simulink model "HIL_Testing_SW_amantest"  (Simulink 7.5)
settings: Solver=ode1  StartTime=0.0  StopTime=Inf  FixedStep=0.001  RelTol=1e-3
PostLoadFcn:
  | , if any(exist('dsrtsu_mdlpostloadfcn', 'file') == [2, 3, 6]), try dsrtsu_mdlpostloadfcn('Execute', bdroot); catch fprintf('Error in PostLoadFcn (dsrtsu_mdlpostloadfcn) for model "%s":\n %s\n', bdroot, lasterr); end, end,
undefined symbols (not defined in the file): CeBSER_Cnt_NumTempAxisPts, ChargeCord, ChargeCord_Control, ChargeToSOCCurr, ChrgCurrLim, CrntSens1Fine, CS_SOCSetPt, CyclerMaxChrgPwr, CyclerMaxDschrgPwr, deltaAhr, Drive_1, Drive_10, Drive_11, Drive_12, Drive_13, Drive_14, Drive_15, Drive_16, Drive_17, Drive_18, Drive_19, Drive_2, Drive_20, Drive_21, Drive_22, Drive_23, Drive_24, Drive_25, Drive_26, Drive_27, Drive_28, Drive_29, Drive_3, Drive_30, Drive_31, Drive_32, Drive_33, Drive_34, Drive_35, Drive_36, Drive_37, Drive_38, Drive_39, Drive_4, Drive_40, Drive_41, Drive_42, Drive_43, Drive_44, Drive_45, Drive_46, Drive_47, Drive_48, Drive_49, Drive_5, Drive_50, Drive_51, Drive_6, Drive_7, Drive_8 ... (+50)
libraries: simulink x129, rtican x50, rti2211sailib x5, rti2211serlib x5, rti2202miolib x3
(part 9 of 23)

== system HIL_Testing_SW_amantest/RX/Read EREV/Read HVEM ==
  Compare To Constant : simulink/Logic and Bit Operations/Compare To Constant  SystemSampleTime=-1  relop=<=  const=0  LogicOutDataTypeMode=uint8  ZeroCross=off
  Current : Subsystem
  Enabled Subsystem : Subsystem  TreatAsAtomicUnit=on
  HV_Battery_Sensed_Output_HV1 : rtican/RTICAN Receive (RX)   SystemSampleTime=-1  Reserved1=[]  Reserved2=[]  Reserved3=[]  Reserved4=[]  SfcnMessage=[]  Msg_Struct=[]  BoardTypeNo=[]  BoardNo=[]  ChannelNo=[]  Parameters=[]  DialogFcn=[]  UnitName=[]  Revision=[]  UnitValues=[]  DSProperties=struct('RTI',struct('Version',uint32(5),'BlockType',struct('isSLSource',uint8(1),'isSLSink',uint8(1),'isHWSource',uint8(0),'isHWSink',uint8(0),'isSetup',uint8(0),'isInline',uint8(1),'isNonInline',uint8(0),'isInterrupt',uint8(0),'isChannelwise',uint8(0)),'IOBoardType','RTICAN','UnitType','MESSAGE','Identifier','RX','DialogType','MSVC','BlockSet','RTICAN','SlaveProcessor','CAN'))  RTIBlockInterface=struct('OutputPortsWidth',int32([1 1 1 1 1 1 1 1 1]),'OutputPortsActive',[1 1 1 1 1 1 1 1 1],'OutputPortsName',{{'HVBSO_Sns2Crnt','HVBSO_Sns1Crnt','HVBSO_BattVltg','HVBSO_Sns2CrntM','HVBSO_Sns1CrntM','HVBSO_BattVltgM','HVBSO_Sns2CrntV','HVBSO_Sns1CrntV','HVBSO_BattVltgV'}},'OutputPortsDataType',{{'SS_DOUBLE','SS_DOUBLE','SS_DOUBLE','SS_DOUBLE','SS_DOUBLE','SS_DOUBLE','SS_DOUBLE','SS_DOUBLE','SS_DOUBLE'}},'OutputPortsLabel',{{'HVBSO_Sns2Crnt','HVBSO_Sns1Crnt','HVBSO_BattVltg','HVBSO_Sns2CrntM','HVBSO_Sns1CrntM','HVBSO_BattVltgM','HVBSO_Sns2CrntV','HVBSO_Sns1CrntV','HVBSO_BattVltgV'}},'OutputPortsLabelMode','ON','InputPortsWidth',int32(0),'InputPortsActive',0,'DialogFcn','rtican_message_interface_gui','BlockDisplay',{{'','center'}},'IconTransparency','on','ParameterTunableNames',{{}},'InitLevel',3,'BlockName',struct('Token',{{'HV_Battery_Sensed_Output_HV'}}),'SampleTime',{{-1}},'TriggerPort',{{'none'}},'EnablePort',{{'none'}})  RTIBlockParameters=struct('BoardTypeNo',{{4302,'OFF',[]}},'BoardNo',{{1,'ON',[1 16]}},'ChannelNo',{{4,'ON',[1 4]}},'Parameters',{{struct('DataFileSupport',struct('DataFileSelectedMaster',1,'DataFileSelectedLocal',1,'DataFileName',['c:\data\databases\6.4.1\globala - hv.dbc|c:\users\hybriderevdomainga\models3x\serialdatabases\v4.4.5(10505)\globala - hvdmx112.dbc|'],'DataFileDate',['04-Jan-2013 08:37:04'],'SelectedFile',['..\databases\8.0.1 (13015)\globala - hv.dbc'],'InterfaceFcn','rtican_dbc_file_parser'),'Options',struct('StatusSelected',0,'TimeSelected',0,'DeltaTimeSelected',0,'BytePortSelected',0,'MessageLengthSelected',0,'TriggerPort',struct('Selected',0,'TriggerType',0),'UserCoding',struct('Selected',0,'InterfaceFile','UserDecodingFile','FcnName','UserDecodeFcn','InportSelected',0,'InportWidth',1,'OutportSelected',0,'OutportWidth',1),'EnablePortSelected',0,'SignalOnPortnameSelected',1,'UseRXService',0),'Message',struct('MsgOnBlocknameSelected',1,'MsgName','HV_Battery_Sensed_Output_HV','MsgIdFormat',0,'MsgId',534,'MsgLength',7,'NumSignals',9,'SampleTime',-1,'Signal',struct('SgnName',{'HVBSO_Sns2Crnt','HVBSO_Sns1Crnt','HVBSO_BattVltg','HVBSO_Sns2CrntM','HVBSO_Sns1CrntM','HVBSO_BattVltgM','HVBSO_Sns2CrntV','HVBSO_Sns1CrntV','HVBSO_BattVltgV'},'SgnStartBit',{0,16,32,44,45,46,47,48,49},'SgnLength',{16,16,12,1,1,1,1,1,1},'ByteLayout',{2,2,2,2,2,2,2,2,2},'Factor',{0.02,0.02,0.125,1,1,1,1,1,1},'Offset',{0,0,0,0,0,0,0,0,0},'SgnComment',{'','','','','','','','',''},'SgnUnit',{'amps','amps','volts','','','','','',''},'Min',{-655.36,-655.36,0,0,0,0,0,0,0},'Max',{655.34,655.34,511.875,1,1,1,1,1,1},'SgnType',{0,0,0,0,0,0,0,0,0},'SLDataType',{'SS_DOUBLE','SS_DOUBLE','SS_DOUBLE','SS_DOUBLE','SS_DOUBLE','SS_DOUBLE','SS_DOUBLE','SS_DOUBLE','SS_DOUBLE'},'DataType',{1,1,0,0,0,0,0,0,0},'ModeValue',{-1,-1,-1,-1,-1,-1,-1,-1,-1}),'MsgIdNumFormat',0,'MsgComment',{{''}}),'Version',1.2,'general',struct('isFromLib',0)),'OFF',[]}},'GroupId',{{struct('Group',{{'RTICAN'}},'No',7,'Behavior',{{'NAMECHANGE'}},'BlockType',{{'SINK'}},'NameChangeFlag',0),'OFF',[]}},'SFcnRTICANMessage',{{struct('MsgType','RX','SFcnPortType','Scalar','MsgName','HV_Battery_Sensed_Output_HV','MsgIdFormat','STD','MsgId',534,'MsgLength',7,'NumSignals',9,'SampleTime',-1,'Signal',struct('SgnName',{'HVBSO_Sns2Crnt','HVBSO_Sns1Crnt','HVBSO_BattVltg','HVBSO_Sns2CrntM','HVBSO_Sns1CrntM','HVBSO_BattVltgM','HVBSO_Sns2CrntV','HVBSO_Sns1CrntV','HVBSO_BattVltgV'},'SgnStartBit',{0,16,32,44,45,46,47,48,49},'SgnLength',{16,16,12,1,1,1,1,1,1},'ByteLayout',{['motorola back.'],['motorola back.'],['motorola back.'],['motorola back.'],['motorola back.'],['motorola back.'],['motorola back.'],['motorola back.'],['motorola back.']},'Factor',{0.02,0.02,0.125,1,1,1,1,1,1},'Offset',{0,0,0,0,0,0,0,0,0},'SgnType',{'standard','standard','standard','standard','standard','standard','standard','standard','standard'},'SLDataType',{'SS_DOUBLE','SS_DOUBLE','SS_DOUBLE','SS_DOUBLE','SS_DOUBLE','SS_DOUBLE','SS_DOUBLE','SS_DOUBLE','SS_DOUBLE'},'DataType',{['signed int'],['signed int'],['unsigned int'],['unsigned int'],['unsigned int'],['unsigned int'],['unsigned int'],['unsigned int'],['unsigned int']},'ModeValue',{-1,-1,-1,-1,-1,-1,-1,-1,-1}),'StatusSelected','no','TimeSelected','no','DeltaTimeSelected','no','BytePortSelected','no','MessageLengthSelected','no','TriggerPort',struct('Selected','no','TriggerType',0),'UserCoding',struct('Selected','no','InterfaceFile','UserDecodingFile','FcnName','UserDecodeFcn','InportSelected','no','InportWidth',1,'OutportSelected','no','OutportWidth',1),'EnablePortSelected','no','UseRXService','no','BoardType','DS4302','BoardNo',1,'ControllerNo',4),'OFF',[]}},'TLCFileName',{{'rtican_rx_message','OFF',[]}})  RTISFcnParameters=struct('SFcnRTICANMessage','struct','TLCFileName','char')  RTIBlockParaDefault=struct('BoardTypeNo',4302,'BoardNo',1,'ChannelNo',1,'Parameters',struct('DataFileSupport',struct('DataFileSelectedMaster',0,'DataFileSelectedLocal',0,'DataFileName','','DataFileDate','','SelectedFile',['<no file selected>']),'Options',struct('StatusSelected',1,'TimeSelected',1,'DeltaTimeSelected',1,'BytePortSelected',0,'MessageLengthSelected',0,'TriggerPort',struct('Selected',0,'TriggerType','rising'),'UserCoding',struct('Selected',0,'InterfaceFile','UserDecodingFile','FcnName','UserDecodeFcn','InportSelected',0,'InportWidth',1,'OutportSelected',0,'OutportWidth',1),'EnablePortSelected',0,'SignalOnPortnameSelected',1,'UseRXService',0),'Message',struct('MsgOnBlocknameSelected',0,'MsgName',['RX Message'],'MsgIdFormat',0,'MsgId',100,'MsgLength',8,'NumSignals',1,'SampleTime',-1,'Signal',struct('SgnName',['RX signal'],'SgnStartBit',0,'SgnLength',8,'SgnType',0,'ModeValue',-1,'DataType',0,'SLDataType','SS_DOUBLE','ByteLayout',0,'Factor',1,'Offset',0,'Min',0,'Max',255,'SgnComment',{{}},'SgnUnit',''),'MsgIdNumFormat',0,'MsgComment',{{''}}),'Version',1.2,'general',struct('isFromLib',1)),'GroupId',struct('Group',{{'RTICAN'}},'No',1,'Behavior',{{'NAMECHANGE'}},'BlockType',{{'SINK'}},'NameChangeFlag',0),'SFcnRTICANMessage',struct('MsgType','RX','MsgName',['RX Message'],'MsgIdFormat','STD','MsgId',100,'MsgLength',8,'NumSignals',1,'SampleTime',-1,'Signal',struct('SgnName',['RX signal'],'SgnStartBit',0,'SgnLength',8,'SgnType','standard','ModeValue',-1,'DataType',['unsigned int'],'ByteLayout',['little endian'],'SLDataType','SS_DOUBLE','Factor',1,'Offset',0),'StatusSelected','yes','TimeSelected','yes','DeltaTimeSelected','yes','BytePortSelected','no','MessageLengthSelected','no','EnablePortSelected','no','UserCoding',struct('Selected','no','InterfaceFile','UserDecodingFile','FcnName','UserDecodeFcn','InportSelected','no','InportWidth',1,'OutportSelected','no','OutportWidth',1),'TriggerPort',struct('Selected','no','TriggerType','rising'),'UseRXService','no','BoardType','DS4302','BoardNo',1,'ControllerNo',1,'SFcnPortType','Scalar'),'TLCFileName','rtican_rx_message')
      settings: AttributesFormatString=Group Id: RTICAN7\n
  High_V_Batt_Temp_Mtrx_HV1 : rtican/RTICAN Receive (RX)   SystemSampleTime=-1  Reserved1=[]  Reserved2=[]  Reserved3=[]  Reserved4=[]  SfcnMessage=[]  Msg_Struct=[]  BoardTypeNo=[]  BoardNo=[]  ChannelNo=[]  Parameters=[]  DialogFcn=[]  UnitName=[]  Revision=[]  UnitValues=[]  DSProperties=struct('RTI',struct('Version',uint32(5),'BlockType',struct('isSLSource',uint8(1),'isSLSink',uint8(1),'isHWSource',uint8(0),'isHWSink',uint8(0),'isSetup',uint8(0),'isInline',uint8(1),'isNonInline',uint8(0),'isInterrupt',uint8(0),'isChannelwise',uint8(0)),'IOBoardType','RTICAN','UnitType','MESSAGE','Identifier','RX','DialogType','MSVC','BlockSet','RTICAN','SlaveProcessor','CAN'))  RTIBlockInterface=struct('OutputPortsWidth',int32([1 1 1 1 1 1 1 1 1 1 1 1 1 1 1 1 1 1 1]),'OutputPortsActive',[1 1 1 1 1 1 1 1 1 1 1 1 1 1 1 1 1 1 1],'OutputPortsName',{{'HVBTMWM_TmpSnFM','HVBTMWM_TmpSnEM','HVBTMWM_TmpSDM','HVBTMWM_TmpSnCM','HVBTMWM_SnIndx','HVBTMWM_TmpSnF','HVBTMWM_TmpSnE','HVBTMWM_TmpSnD','HVBTMWM_TmpSnC','HVBTMWM_TmpSnB','HVBTMWM_TmpSnA','HVBTMWM_TmpSnBM','HVBTMWM_TmpSnAM','HVBTMWM_TmpSnFV','HVBTMWM_TmpSnEV','HVBTMWM_TmpSnDV','HVBTMWM_TmpSnCV','HVBTMWM_TmpSnBV','HVBTMWM_TmpSnAV'}},'OutputPortsDataType',{{'SS_DOUBLE','SS_DOUBLE','SS_DOUBLE','SS_DOUBLE','SS_DOUBLE','SS_DOUBLE','SS_DOUBLE','SS_DOUBLE','SS_DOUBLE','SS_DOUBLE','SS_DOUBLE','SS_DOUBLE','SS_DOUBLE','SS_DOUBLE','SS_DOUBLE','SS_DOUBLE','SS_DOUBLE','SS_DOUBLE','SS_DOUBLE'}},'OutputPortsLabel',{{'HVBTMWM_TmpSnFM','HVBTMWM_TmpSnEM','HVBTMWM_TmpSDM','HVBTMWM_TmpSnCM','HVBTMWM_SnIndx','HVBTMWM_TmpSnF','HVBTMWM_TmpSnE','HVBTMWM_TmpSnD','HVBTMWM_TmpSnC','HVBTMWM_TmpSnB','HVBTMWM_TmpSnA','HVBTMWM_TmpSnBM','HVBTMWM_TmpSnAM','HVBTMWM_TmpSnFV','HVBTMWM_TmpSnEV','HVBTMWM_TmpSnDV','HVBTMWM_TmpSnCV','HVBTMWM_TmpSnBV','HVBTMWM_TmpSnAV'}},'OutputPortsLabelMode','ON','InputPortsWidth',int32(0),'InputPortsActive',0,'DialogFcn','rtican_message_interface_gui','BlockDisplay',{{'','center'}},'IconTransparency','on','ParameterTunableNames',{{}},'InitLevel',3,'BlockName',struct('Token',{{'High_V_Batt_Temp_Mtrx_HV'}}),'SampleTime',{{-1}},'TriggerPort',{{'none'}},'EnablePort',{{'none'}})  RTIBlockParameters=struct('BoardTypeNo',{{4302,'OFF',[]}},'BoardNo',{{1,'ON',[1 16]}},'ChannelNo',{{4,'ON',[1 4]}},'Parameters',{{struct('DataFileSupport',struct('DataFileSelectedMaster',1,'DataFileSelectedLocal',1,'DataFileName',['c:\data\databases\6.4.1\globala - hv.dbc|c:\users\hybriderevdomainga\models3x\serialdatabases\v4.4.5(10505)\globala - hvdmx112.dbc|'],'DataFileDate',['04-Jan-2013 08:37:04'],'SelectedFile',['..\databases\8.0.1 (13015)\globala - hv.dbc'],'InterfaceFcn','rtican_dbc_file_parser'),'Options',struct('StatusSelected',0,'TimeSelected',0,'DeltaTimeSelected',0,'BytePortSelected',0,'MessageLengthSelected',0,'TriggerPort',struct('Selected',0,'TriggerType',0),'UserCoding',struct('Selected',0,'InterfaceFile','UserDecodingFile','FcnName','UserDecodeFcn','InportSelected',0,'InportWidth',1,'OutportSelected',0,'OutportWidth',1),'EnablePortSelected',0,'SignalOnPortnameSelected',1,'UseRXService',0),'Message',struct('MsgOnBlocknameSelected',1,'MsgName','High_V_Batt_Temp_Mtrx_HV','MsgIdFormat',0,'MsgId',770,'MsgLength',8,'NumSignals',19,'SampleTime',-1,'Signal',struct('SgnName',{'HVBTMWM_TmpSnFM','HVBTMWM_TmpSnEM','HVBTMWM_TmpSDM','HVBTMWM_TmpSnCM','HVBTMWM_SnIndx','HVBTMWM_TmpSnF','HVBTMWM_TmpSnE','HVBTMWM_TmpSnD','HVBTMWM_TmpSnC','HVBTMWM_TmpSnB','HVBTMWM_TmpSnA','HVBTMWM_TmpSnBM','HVBTMWM_TmpSnAM','HVBTMWM_TmpSnFV','HVBTMWM_TmpSnEV','HVBTMWM_TmpSnDV','HVBTMWM_TmpSnCV','HVBTMWM_TmpSnBV','HVBTMWM_TmpSnAV'},'SgnStartBit',{1,2,3,4,5,8,16,24,32,40,48,56,57,58,59,60,61,62,63},'SgnLength',{1,1,1,1,3,8,8,8,8,8,8,1,1,1,1,1,1,1,1},'ByteLayout',{2,2,2,2,2,2,2,2,2,2,2,2,2,2,2,2,2,2,2},'Factor',{1,1,1,1,1,0.5,0.5,0.5,0.5,0.5,0.5,1,1,1,1,1,1,1,1},'Offset',{0,0,0,0,0,-40,-40,-40,-40,-40,-40,0,0,0,0,0,0,0,0},'SgnComment',{'','','','','','','','','','','','','','','','','','',''},'SgnUnit',{'','','','','',['deg C'],['deg C'],['deg C'],['deg C'],['deg C'],['deg C'],'','','','','','','',''},'Min',{0,0,0,0,0,-40,-40,-40,-40,-40,-40,0,0,0,0,0,0,0,0},'Max',{1,1,1,1,7,87.5,87.5,87.5,87.5,87.5,87.5,1,1,1,1,1,1,1,1},'SgnType',{0,0,0,0,0,0,0,0,0,0,0,0,0,0,0,0,0,0,0},'SLDataType',{'SS_DOUBLE','SS_DOUBLE','SS_DOUBLE','SS_DOUBLE','SS_DOUBLE','SS_DOUBLE','SS_DOUBLE','SS_DOUBLE','SS_DOUBLE','SS_DOUBLE','SS_DOUBLE','SS_DOUBLE','SS_DOUBLE','SS_DOUBLE','SS_DOUBLE','SS_DOUBLE','SS_DOUBLE','SS_DOUBLE','SS_DOUBLE'},'DataType',{0,0,0,0,0,0,0,0,0,0,0,0,0,0,0,0,0,0,0},'ModeValue',{-1,-1,-1,-1,-1,-1,-1,-1,-1,-1,-1,-1,-1,-1,-1,-1,-1,-1,-1}),'MsgIdNumFormat',0,'MsgComment',{{''}}),'Version',1.2,'general',struct('isFromLib',0)),'OFF',[]}},'GroupId',{{struct('Group',{{'RTICAN'}},'No',7,'Behavior',{{'NAMECHANGE'}},'BlockType',{{'SINK'}},'NameChangeFlag',0),'OFF',[]}},'SFcnRTICANMessage',{{struct('MsgType','RX','SFcnPortType','Scalar','MsgName','High_V_Batt_Temp_Mtrx_HV','MsgIdFormat','STD','MsgId',770,'MsgLength',8,'NumSignals',19,'SampleTime',-1,'Signal',struct('SgnName',{'HVBTMWM_TmpSnFM','HVBTMWM_TmpSnEM','HVBTMWM_TmpSDM','HVBTMWM_TmpSnCM','HVBTMWM_SnIndx','HVBTMWM_TmpSnF','HVBTMWM_TmpSnE','HVBTMWM_TmpSnD','HVBTMWM_TmpSnC','HVBTMWM_TmpSnB','HVBTMWM_TmpSnA','HVBTMWM_TmpSnBM','HVBTMWM_TmpSnAM','HVBTMWM_TmpSnFV','HVBTMWM_TmpSnEV','HVBTMWM_TmpSnDV','HVBTMWM_TmpSnCV','HVBTMWM_TmpSnBV','HVBTMWM_TmpSnAV'},'SgnStartBit',{1,2,3,4,5,8,16,24,32,40,48,56,57,58,59,60,61,62,63},'SgnLength',{1,1,1,1,3,8,8,8,8,8,8,1,1,1,1,1,1,1,1},'ByteLayout',{['motorola back.'],['motorola back.'],['motorola back.'],['motorola back.'],['motorola back.'],['motorola back.'],['motorola back.'],['motorola back.'],['motorola back.'],['motorola back.'],['motorola back.'],['motorola back.'],['motorola back.'],['motorola back.'],['motorola back.'],['motorola back.'],['motorola back.'],['motorola back.'],['motorola back.']},'Factor',{1,1,1,1,1,0.5,0.5,0.5,0.5,0.5,0.5,1,1,1,1,1,1,1,1},'Offset',{0,0,0,0,0,-40,-40,-40,-40,-40,-40,0,0,0,0,0,0,0,0},'SgnType',{'standard','standard','standard','standard','standard','standard','standard','standard','standard','standard','standard','standard','standard','standard','standard','standard','standard','standard','standard'},'SLDataType',{'SS_DOUBLE','SS_DOUBLE','SS_DOUBLE','SS_DOUBLE','SS_DOUBLE','SS_DOUBLE','SS_DOUBLE','SS_DOUBLE','SS_DOUBLE','SS_DOUBLE','SS_DOUBLE','SS_DOUBLE','SS_DOUBLE','SS_DOUBLE','SS_DOUBLE','SS_DOUBLE','SS_DOUBLE','SS_DOUBLE','SS_DOUBLE'},'DataType',{['unsigned int'],['unsigned int'],['unsigned int'],['unsigned int'],['unsigned int'],['unsigned int'],['unsigned int'],['unsigned int'],['unsigned int'],['unsigned int'],['unsigned int'],['unsigned int'],['unsigned int'],['unsigned int'],['unsigned int'],['unsigned int'],['unsigned int'],['unsigned int'],['unsigned int']},'ModeValue',{-1,-1,-1,-1,-1,-1,-1,-1,-1,-1,-1,-1,-1,-1,-1,-1,-1,-1,-1}),'StatusSelected','no','TimeSelected','no','DeltaTimeSelected','no','BytePortSelected','no','MessageLengthSelected','no','TriggerPort',struct('Selected','no','TriggerType',0),'UserCoding',struct('Selected','no','InterfaceFile','UserDecodingFile','FcnName','UserDecodeFcn','InportSelected','no','InportWidth',1,'OutportSelected','no','OutportWidth',1),'EnablePortSelected','no','UseRXService','no','BoardType','DS4302','BoardNo',1,'ControllerNo',4),'OFF',[]}},'TLCFileName',{{'rtican_rx_message','OFF',[]}})  RTISFcnParameters=struct('SFcnRTICANMessage','struct','TLCFileName','char')  RTIBlockParaDefault=struct('BoardTypeNo',4302,'BoardNo',1,'ChannelNo',1,'Parameters',struct('DataFileSupport',struct('DataFileSelectedMaster',0,'DataFileSelectedLocal',0,'DataFileName','','DataFileDate','','SelectedFile',['<no file selected>']),'Options',struct('StatusSelected',1,'TimeSelected',1,'DeltaTimeSelected',1,'BytePortSelected',0,'MessageLengthSelected',0,'TriggerPort',struct('Selected',0,'TriggerType','rising'),'UserCoding',struct('Selected',0,'InterfaceFile','UserDecodingFile','FcnName','UserDecodeFcn','InportSelected',0,'InportWidth',1,'OutportSelected',0,'OutportWidth',1),'EnablePortSelected',0,'SignalOnPortnameSelected',1,'UseRXService',0),'Message',struct('MsgOnBlocknameSelected',0,'MsgName',['RX Message'],'MsgIdFormat',0,'MsgId',100,'MsgLength',8,'NumSignals',1,'SampleTime',-1,'Signal',struct('SgnName',['RX signal'],'SgnStartBit',0,'SgnLength',8,'SgnType',0,'ModeValue',-1,'DataType',0,'SLDataType','SS_DOUBLE','ByteLayout',0,'Factor',1,'Offset',0,'Min',0,'Max',255,'SgnComment',{{}},'SgnUnit',''),'MsgIdNumFormat',0,'MsgComment',{{''}}),'Version',1.2,'general',struct('isFromLib',1)),'GroupId',struct('Group',{{'RTICAN'}},'No',1,'Behavior',{{'NAMECHANGE'}},'BlockType',{{'SINK'}},'NameChangeFlag',0),'SFcnRTICANMessage',struct('MsgType','RX','MsgName',['RX Message'],'MsgIdFormat','STD','MsgId',100,'MsgLength',8,'NumSignals',1,'SampleTime',-1,'Signal',struct('SgnName',['RX signal'],'SgnStartBit',0,'SgnLength',8,'SgnType','standard','ModeValue',-1,'DataType',['unsigned int'],'ByteLayout',['little endian'],'SLDataType','SS_DOUBLE','Factor',1,'Offset',0),'StatusSelected','yes','TimeSelected','yes','DeltaTimeSelected','yes','BytePortSelected','no','MessageLengthSelected','no','EnablePortSelected','no','UserCoding',struct('Selected','no','InterfaceFile','UserDecodingFile','FcnName','UserDecodeFcn','InportSelected','no','InportWidth',1,'OutportSelected','no','OutportWidth',1),'TriggerPort',struct('Selected','no','TriggerType','rising'),'UseRXService','no','BoardType','DS4302','BoardNo',1,'ControllerNo',1,'SFcnPortType','Scalar'),'TLCFileName','rtican_rx_message')
      settings: AttributesFormatString=Group Id: RTICAN7\n
  Sum of Cells : Subsystem
  Terminator{1..11,19,22..29,33..36,52..54,58..59} (29 alike) : Terminator
  VICM_Status_HV : rtican/RTICAN Receive (RX)   SystemSampleTime=-1  Reserved1=[]  Reserved2=[]  Reserved3=[]  Reserved4=[]  SfcnMessage=[]  Msg_Struct=[]  BoardTypeNo=[]  BoardNo=[]  ChannelNo=[]  Parameters=[]  DialogFcn=[]  UnitName=[]  Revision=[]  UnitValues=[]  DSProperties=struct('RTI',struct('Version',uint32(5),'BlockType',struct('isSLSource',uint8(1),'isSLSink',uint8(1),'isHWSource',uint8(0),'isHWSink',uint8(0),'isSetup',uint8(0),'isInline',uint8(1),'isNonInline',uint8(0),'isInterrupt',uint8(0),'isChannelwise',uint8(0)),'IOBoardType','RTICAN','UnitType','MESSAGE','Identifier','RX','DialogType','MSVC','BlockSet','RTICAN','SlaveProcessor','CAN'))  RTIBlockInterface=struct('OutputPortsWidth',int32([1 1 1 1 1 1 1 1 1 1 1 1]),'OutputPortsActive',[1 1 1 1 1 1 1 1 1 1 1 1],'OutputPortsName',{{'CstmrUsblSOC','VehEnrgyReq','VehEnrgyCap','HVBtClOVFFTstRq','HVBatLwParMdReq','ChrgrPmpPrcntSpd','ChrgrPmpEnbl','HVBtClOVFFTstIdx','ChrgrCntctrStatus','HVCntctrStat','VICntlModRunCrkTrmSt','VICMClrLgsDgInfo'}},'OutputPortsDataType',{{'SS_DOUBLE','SS_DOUBLE','SS_DOUBLE','SS_DOUBLE','SS_DOUBLE','SS_DOUBLE','SS_DOUBLE','SS_DOUBLE','SS_DOUBLE','SS_DOUBLE','SS_DOUBLE','SS_DOUBLE'}},'OutputPortsLabel',{{'CstmrUsblSOC','VehEnrgyReq','VehEnrgyCap','HVBtClOVFFTstRq','HVBatLwParMdReq','ChrgrPmpPrcntSpd','ChrgrPmpEnbl','HVBtClOVFFTstIdx','ChrgrCntctrStatus','HVCntctrStat','VICntlModRunCrkTrmSt','VICMClrLgsDgInfo'}},'OutputPortsLabelMode','ON','InputPortsWidth',int32(0),'InputPortsActive',0,'DialogFcn','rtican_message_interface_gui','BlockDisplay',{{'','center'}},'IconTransparency','on','ParameterTunableNames',{{}},'InitLevel',3,'BlockName',struct('Token',{{'VICM_Status_HV'}}),'SampleTime',{{-1}},'TriggerPort',{{'none'}},'EnablePort',{{'none'}})  RTIBlockParameters=struct('BoardTypeNo',{{4302,'OFF',[]}},'BoardNo',{{1,'ON',[1 16]}},'ChannelNo',{{4,'ON',[1 4]}},'Parameters',{{struct('DataFileSupport',struct('DataFileSelectedMaster',1,'DataFileSelectedLocal',1,'DataFileName',['c:\data\databases\8.0.1 (13015)\globala - hv.dbc|c:\data\testing\dbc\globala - hvdmx112.dbc|'],'DataFileDate',['04-Jan-2013 08:37:04'],'SelectedFile',['..\databases\8.0.1 (13015)\globala - hv.dbc'],'InterfaceFcn','rtican_dbc_file_parser'),'Options',struct('StatusSelected',0,'TimeSelected',0,'DeltaTimeSelected',0,'BytePortSelected',0,'MessageLengthSelected',0,'TriggerPort',struct('Selected',0,'TriggerType',0),'UserCoding',struct('Selected',0,'InterfaceFile','UserDecodingFile','FcnName','UserDecodeFcn','InportSelected',0,'InportWidth',1,'OutportSelected',0,'OutportWidth',1),'EnablePortSelected',0,'SignalOnPortnameSelected',1,'UseRXService',0),'Message',struct('MsgOnBlocknameSelected',1,'MsgName','VICM_Status_HV','MsgIdFormat',0,'MsgId',522,'MsgLength',8,'NumSignals',12,'SampleTime',-1,'Signal',struct('SgnName',{'CstmrUsblSOC','VehEnrgyReq','VehEnrgyCap','HVBtClOVFFTstRq','HVBatLwParMdReq','ChrgrPmpPrcntSpd','ChrgrPmpEnbl','HVBtClOVFFTstIdx','ChrgrCntctrStatus','HVCntctrStat','VICntlModRunCrkTrmSt','VICMClrLgsDgInfo'},'SgnStartBit',{0,8,24,38,39,40,48,49,56,59,62,63},'SgnLength',{8,16,14,1,1,8,1,7,3,3,1,1},'SgnType',{0,0,0,0,0,0,0,0,0,0,0,0},'ModeValue',{-1,-1,-1,-1,-1,-1,-1,-1,-1,-1,-1,-1},'DataType',{0,0,0,0,0,0,0,0,0,0,0,0},'ByteLayout',{2,2,2,2,2,2,2,2,2,2,2,2},'Factor',{0.39216,0.36,0.36,1,1,0.392157,1,1,1,1,1,1},'Offset',{0,0,3.6,0,0,0,0,0,0,0,0,0},'SgnComment',{{''},{''},{''},{''},{''},{''},{''},{''},{''},{''},{''},{''}},'SgnUnit',{'%','MJ','MJ','','','%','','','','','',''},'Min',{0,0,3.6,0,0,0,0,0,0,0,0,0},'Max',{100.0008,23592.6,5901.48,1,1,100.000035,1,127,7,7,1,1},'SLDataType',{'SS_DOUBLE','SS_DOUBLE','SS_DOUBLE','SS_DOUBLE','SS_DOUBLE','SS_DOUBLE','SS_DOUBLE','SS_DOUBLE','SS_DOUBLE','SS_DOUBLE','SS_DOUBLE','SS_DOUBLE'}),'MsgIdNumFormat',0,'MsgComment',{{''}}),'Version',1.2,'general',struct('isFromLib',0)),'OFF',[]}},'GroupId',{{struct('Group',{{'RTICAN'}},'No',7,'Behavior',{{'NAMECHANGE'}},'BlockType',{{'SINK'}},'NameChangeFlag',0),'OFF',[]}},'SFcnRTICANMessage',{{struct('MsgType','RX','SFcnPortType','Scalar','MsgName','VICM_Status_HV','MsgIdFormat','STD','MsgId',522,'MsgLength',8,'NumSignals',12,'SampleTime',-1,'Signal',struct('SgnName',{'CstmrUsblSOC','VehEnrgyReq','VehEnrgyCap','HVBtClOVFFTstRq','HVBatLwParMdReq','ChrgrPmpPrcntSpd','ChrgrPmpEnbl','HVBtClOVFFTstIdx','ChrgrCntctrStatus','HVCntctrStat','VICntlModRunCrkTrmSt','VICMClrLgsDgInfo'},'SgnStartBit',{0,8,24,38,39,40,48,49,56,59,62,63},'SgnLength',{8,16,14,1,1,8,1,7,3,3,1,1},'SgnType',{'standard','standard','standard','standard','standard','standard','standard','standard','standard','standard','standard','standard'},'ModeValue',{-1,-1,-1,-1,-1,-1,-1,-1,-1,-1,-1,-1},'DataType',{['unsigned int'],['unsigned int'],['unsigned int'],['unsigned int'],['unsigned int'],['unsigned int'],['unsigned int'],['unsigned int'],['unsigned int'],['unsigned int'],['unsigned int'],['unsigned int']},'ByteLayout',{['motorola back.'],['motorola back.'],['motorola back.'],['motorola back.'],['motorola back.'],['motorola back.'],['motorola back.'],['motorola back.'],['motorola back.'],['motorola back.'],['motorola back.'],['motorola back.']},'Factor',{0.39216,0.36,0.36,1,1,0.392157,1,1,1,1,1,1},'Offset',{0,0,3.6,0,0,0,0,0,0,0,0,0},'SLDataType',{'SS_DOUBLE','SS_DOUBLE','SS_DOUBLE','SS_DOUBLE','SS_DOUBLE','SS_DOUBLE','SS_DOUBLE','SS_DOUBLE','SS_DOUBLE','SS_DOUBLE','SS_DOUBLE','SS_DOUBLE'}),'StatusSelected','no','TimeSelected','no','DeltaTimeSelected','no','BytePortSelected','no','MessageLengthSelected','no','TriggerPort',struct('Selected','no','TriggerType',0),'UserCoding',struct('Selected','no','InterfaceFile','UserDecodingFile','FcnName','UserDecodeFcn','InportSelected','no','InportWidth',1,'OutportSelected','no','OutportWidth',1),'EnablePortSelected','no','UseRXService','no','BoardType','DS4302','BoardNo',1,'ControllerNo',4),'OFF',[]}},'TLCFileName',{{'rtican_rx_message','OFF',[]}})  RTISFcnParameters=struct('SFcnRTICANMessage','struct','TLCFileName','char')  RTIBlockParaDefault=struct('BoardTypeNo',4302,'BoardNo',1,'ChannelNo',1,'Parameters',struct('DataFileSupport',struct('DataFileSelectedMaster',0,'DataFileSelectedLocal',0,'DataFileName','','DataFileDate','','SelectedFile',['<no file selected>']),'Options',struct('StatusSelected',1,'TimeSelected',1,'DeltaTimeSelected',1,'BytePortSelected',0,'MessageLengthSelected',0,'TriggerPort',struct('Selected',0,'TriggerType','rising'),'UserCoding',struct('Selected',0,'InterfaceFile','UserDecodingFile','FcnName','UserDecodeFcn','InportSelected',0,'InportWidth',1,'OutportSelected',0,'OutportWidth',1),'EnablePortSelected',0,'SignalOnPortnameSelected',1,'UseRXService',0),'Message',struct('MsgOnBlocknameSelected',0,'MsgName',['RX Message'],'MsgIdFormat',0,'MsgId',100,'MsgLength',8,'NumSignals',1,'SampleTime',-1,'Signal',struct('SgnName',['RX signal'],'SgnStartBit',0,'SgnLength',8,'SgnType',0,'ModeValue',-1,'DataType',0,'SLDataType','SS_DOUBLE','ByteLayout',0,'Factor',1,'Offset',0,'Min',0,'Max',255,'SgnComment',{{}},'SgnUnit',''),'MsgIdNumFormat',0,'MsgComment',{{''}}),'Version',1.2,'general',struct('isFromLib',1)),'GroupId',struct('Group',{{'RTICAN'}},'No',1,'Behavior',{{'NAMECHANGE'}},'BlockType',{{'SINK'}},'NameChangeFlag',0),'SFcnRTICANMessage',struct('MsgType','RX','MsgName',['RX Message'],'MsgIdFormat','STD','MsgId',100,'MsgLength',8,'NumSignals',1,'SampleTime',-1,'Signal',struct('SgnName',['RX signal'],'SgnStartBit',0,'SgnLength',8,'SgnType','standard','ModeValue',-1,'DataType',['unsigned int'],'ByteLayout',['little endian'],'SLDataType','SS_DOUBLE','Factor',1,'Offset',0),'StatusSelected','yes','TimeSelected','yes','DeltaTimeSelected','yes','BytePortSelected','no','MessageLengthSelected','no','EnablePortSelected','no','UserCoding',struct('Selected','no','InterfaceFile','UserDecodingFile','FcnName','UserDecodeFcn','InportSelected','no','InportWidth',1,'OutportSelected','no','OutportWidth',1),'TriggerPort',struct('Selected','no','TriggerType','rising'),'UseRXService','no','BoardType','DS4302','BoardNo',1,'ControllerNo',1,'SFcnPortType','Scalar'),'TLCFileName','rtican_rx_message')
      settings: AttributesFormatString=Group Id: RTICAN7\n
  SumOfCells : Outport  OutDataType=sfix(16)  OutScaling=2^0
  MinCell : Outport  Port=2  OutDataType=sfix(16)  OutScaling=2^0
  MaxCell : Outport  Port=3  OutDataType=sfix(16)  OutScaling=2^0
  MinSectionVoltage : Outport  Port=4  OutDataType=sfix(16)  OutScaling=2^0
  HVCntctrStat : Outport  Port=5  OutDataType=sfix(16)  OutScaling=2^0
  PackCurrent : Outport  Port=6  OutDataType=sfix(16)  OutScaling=2^0
  PackVoltage : Outport  Port=7  OutDataType=sfix(16)  OutScaling=2^0
  BatTemp : Outport  Port=8  OutDataType=sfix(16)  OutScaling=2^0
  wires:
  Sum of Cells/2(MinCell) -> MinCell/1  "MinCell"
  Sum of Cells/3(MaxCell) -> MaxCell/1  "MaxCell"
  High_V_Batt_Temp_Mtrx_HV1/1 -> Terminator36/1  "HVBTMWM_TmpSnFM"
  High_V_Batt_Temp_Mtrx_HV1/2 -> Terminator35/1  "HVBTMWM_TmpSnEM"
  High_V_Batt_Temp_Mtrx_HV1/3 -> Terminator34/1  "HVBTMWM_TmpSDM"
  High_V_Batt_Temp_Mtrx_HV1/4 -> Terminator33/1  "HVBTMWM_TmpSnCM"
  High_V_Batt_Temp_Mtrx_HV1/5 -> Compare To Constant/1  "HVBTMWM_SnIndx"
  High_V_Batt_Temp_Mtrx_HV1/6 -> Enabled Subsystem/1(In1)  "HVBTMWM_TmpSnF"
  High_V_Batt_Temp_Mtrx_HV1/7 -> Enabled Subsystem/2(In2)  "HVBTMWM_TmpSnE"
  High_V_Batt_Temp_Mtrx_HV1/8 -> Enabled Subsystem/3(In3)  "HVBTMWM_TmpSnD"
  High_V_Batt_Temp_Mtrx_HV1/9 -> Enabled Subsystem/4(In4)  "HVBTMWM_TmpSnC"
  High_V_Batt_Temp_Mtrx_HV1/10 -> Enabled Subsystem/5(In5)  "HVBTMWM_TmpSnB"
  High_V_Batt_Temp_Mtrx_HV1/11 -> Enabled Subsystem/6(In6)  "HVBTMWM_TmpSnA"
  High_V_Batt_Temp_Mtrx_HV1/12 -> Terminator59/1  "HVBTMWM_TmpSnBM"
  High_V_Batt_Temp_Mtrx_HV1/13 -> Terminator58/1  "HVBTMWM_TmpSnAM"
  High_V_Batt_Temp_Mtrx_HV1/14 -> Terminator52/1  "HVBTMWM_TmpSnFV"
  High_V_Batt_Temp_Mtrx_HV1/15 -> Terminator54/1  "HVBTMWM_TmpSnEV"
  High_V_Batt_Temp_Mtrx_HV1/16 -> Terminator53/1  "HVBTMWM_TmpSnDV"
  High_V_Batt_Temp_Mtrx_HV1/17 -> Terminator4/1  "HVBTMWM_TmpSnCV"
  High_V_Batt_Temp_Mtrx_HV1/18 -> Terminator6/1  "HVBTMWM_TmpSnBV"
  High_V_Batt_Temp_Mtrx_HV1/19 -> Terminator5/1  "HVBTMWM_TmpSnAV"
  Compare To Constant/1 -> Enabled Subsystem/Enable
  HV_Battery_Sensed_Output_HV1/4 -> Terminator19/1  "HVBSO_Sns2CrntM"
  Current/1(Out1) -> PackCurrent/1  "PackCurrent"
  HV_Battery_Sensed_Output_HV1/3 -> PackVoltage/1  "HVBSO_BattVltg"
  VICM_Status_HV/2 -> Terminator22/1  "VehEnrgyReq"
  VICM_Status_HV/3 -> Terminator23/1  "VehEnrgyCap"
  VICM_Status_HV/4 -> Terminator24/1  "HVBtClOVFFTstRq"
  VICM_Status_HV/5 -> Terminator27/1  "HVBatLwParMdReq"
  VICM_Status_HV/6 -> Terminator26/1  "ChrgrPmpPrcntSpd"
  VICM_Status_HV/7 -> Terminator25/1  "ChrgrPmpEnbl"
  VICM_Status_HV/8 -> Terminator28/1  "HVBtClOVFFTstIdx"
  VICM_Status_HV/9 -> Terminator29/1  "ChrgrCntctrStatus"
  VICM_Status_HV/11 -> Terminator2/1  "VICntlModRunCrkTrmSt"
  VICM_Status_HV/12 -> Terminator1/1  "VICMClrLgsDgInfo"
  VICM_Status_HV/1 -> Terminator3/1  "CstmrUsblSOC"
  Sum of Cells/1(SumCells) -> SumOfCells/1
  Sum of Cells/4(MinSection_PackEquivalent) -> MinSectionVoltage/1
  VICM_Status_HV/10 -> HVCntctrStat/1  "HVCntctrStat"
  HV_Battery_Sensed_Output_HV1/1 -> Current/1(SensTwo)  "HVBSO_Sns2Crnt"
  HV_Battery_Sensed_Output_HV1/2 -> Current/2(SensOne)  "HVBSO_Sns1Crnt"
  Enabled Subsystem/1(TempAvg) -> BatTemp/1
  HV_Battery_Sensed_Output_HV1/5 -> Terminator7/1  "HVBSO_Sns1CrntM"
  HV_Battery_Sensed_Output_HV1/6 -> Terminator8/1  "HVBSO_BattVltgM"
  HV_Battery_Sensed_Output_HV1/7 -> Terminator9/1  "HVBSO_Sns2CrntV"
  HV_Battery_Sensed_Output_HV1/8 -> Terminator10/1  "HVBSO_Sns1CrntV"
  HV_Battery_Sensed_Output_HV1/9 -> Terminator11/1  "HVBSO_BattVltgV"
